simulink model "verify_Collector_EN12975_FlatPlate_mdl"  (R2016b)
settings: Solver=ode45  StartTime=0  StopTime=24*3600  MaxStep=600  RelTol=1e-3  EnableMultiTasking=on
InitFcn:
  | load('DE_TRY2010_13_averageYear')
libraries: carnot x4
settings Model: Creator=drhf  LastModifiedBy=User
settings DataIOCC: SaveFormat=Array  SignalLoggingSaveFormat=ModelDataLogs
settings OptimizationCC: ExpressionDepthLimit=2147483647  LifeSpan=inf
settings DebuggingCC: UnderspecifiedInitializationDetection=Classic  MergeDetectMultiDrivingBlocksExec=none  SolverPrmCheckMsg=warning  FcnCallInpInsideContextMsg=warning  StateNameClashWarn=warning  SFUnexpectedBacktrackingDiag=warning  SFNoUnconditionalDefaultTransitionDiag=warning  SFExecutionAtInitializationDiag=none
settings HardwareCC: ProdBitPerPointer=32  ProdBitPerSizeT=32  ProdBitPerPtrDiffT=32  ProdLargestAtomicFloat=None  ProdIntDivRoundTo=Undefined  ProdEndianess=Unspecified  ProdWordSize=32  ProdHWDeviceType=32-bit Generic
settings ModelReferenceCC: PropagateSignalLabelsOutOfModel=off
settings GRTTargetCC: TargetLangStandard=C89/C90 (ANSI)  GeneratePreprocessorConditionals=Disable all  CombineOutputUpdateFcns=off  GRTInterface=on
settings ConfigComp: CovMetricSettings=dw  CovHtmlReporting=on  CovSaveCumulativeToWorkspaceVar=on  CovSaveSingleToWorkspaceVar=on  CovExternalEMLEnable=off

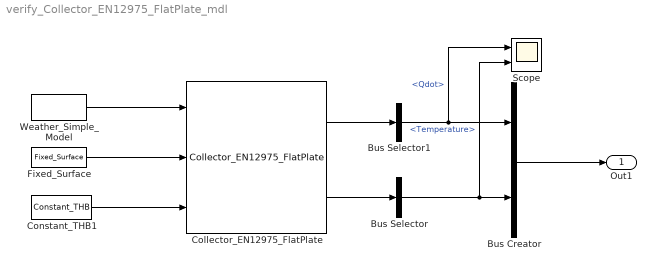
== system verify_Collector_EN12975_FlatPlate_mdl ==
  Bus Creator : BusCreator  Inputs=2
  Bus Selector : BusSelector  OutputSignals=Temperature
  Bus Selector1 : BusSelector  OutputSignals=Qdot
  Collector_EN12975_FlatPlate : carnot/Source/Solar_Thermal/Collector_EN12975_FlatPlate  acol=2.5  len=2.3  fta=0.8103  c1=3.757  c2=0.0147  c3=0  c4=0  c5=7062  c6=0  b0=0.12  Kd=0.92  lin=0  qua=0  tini=20
  Constant_THB1 : carnot/Source/Simple/Constant_THB  t=40  mdot=100/3600  p=1e5  mID=Full Pressure Drop with Static Height  fluid=Water  mix=0  mix2=0  mix3=0  dia=0.02  hgt=0
  Fixed_Surface : carnot/Weather/Fixed_Surface  colangle=30  colazi=0  colrot=0
  Scope : Scope  NumInputPorts=2
  Weather_Simple_Model : carnot/Weather/Weather_Simple_Model  lat=60  Ibn=900  Idg=100  tamb=5  deltaTsky=-6  rh=50  precip="10e-3/24/3600           % 10 mm in 24 h"  cloud=0.125  p=1013e2  vw=1  wdir=270
  Out1 : Outport
  wires:
  Bus Creator/1 -> Out1/1
  Collector_EN12975_FlatPlate/2 -> Bus Selector/1
  Weather_Simple_Model/1 -> Collector_EN12975_FlatPlate/1
  Constant_THB1/1 -> Collector_EN12975_FlatPlate/3
  Fixed_Surface/1 -> Collector_EN12975_FlatPlate/2
  Collector_EN12975_FlatPlate/1 -> Bus Selector1/1
  Bus Selector/1 -> Scope/2, Bus Creator/2  "<Temperature>"
  Bus Selector1/1 -> Scope/1, Bus Creator/1  "<Qdot>"
